simulink model "DSimulator_robot3GDL"  (Simulink 9.0)
settings: Solver=ode1  StartTime=0  StopTime=60  FixedStep=0.004  RelTol=1e-3  EnableMultiTasking=on
undefined symbols (not defined in the file or in its folder): Dinamic_ur10_3DOF, SimpleRobotPlotROS, Tau_JointSpace, Tau_OperationalSpace, TrajGen_JointSpace, TrajGen_OperationalSpace
libraries: simulink x3
settings Model: SuppressorTable=22 serialization::archive 11 0 6 0 0 0 11 0  Creator=E. Dean  LastModifiedBy=nirnai
settings DataIOCC: LimitDataPoints=on  SignalLoggingSaveFormat=ModelDataLogs
settings OptimizationCC: ExpressionDepthLimit=2147483647
settings DebuggingCC: SolverPrmCheckMsg=warning  FcnCallInpInsideContextMsg=warning  AllowSymbolicDim=off  StateNameClashWarn=warning
settings GRTTargetCC: GeneratePreprocessorConditionals=Disable all  CombineOutputUpdateFcns=off  GRTInterface=on
settings ConfigComp: CovSFcnEnable=off

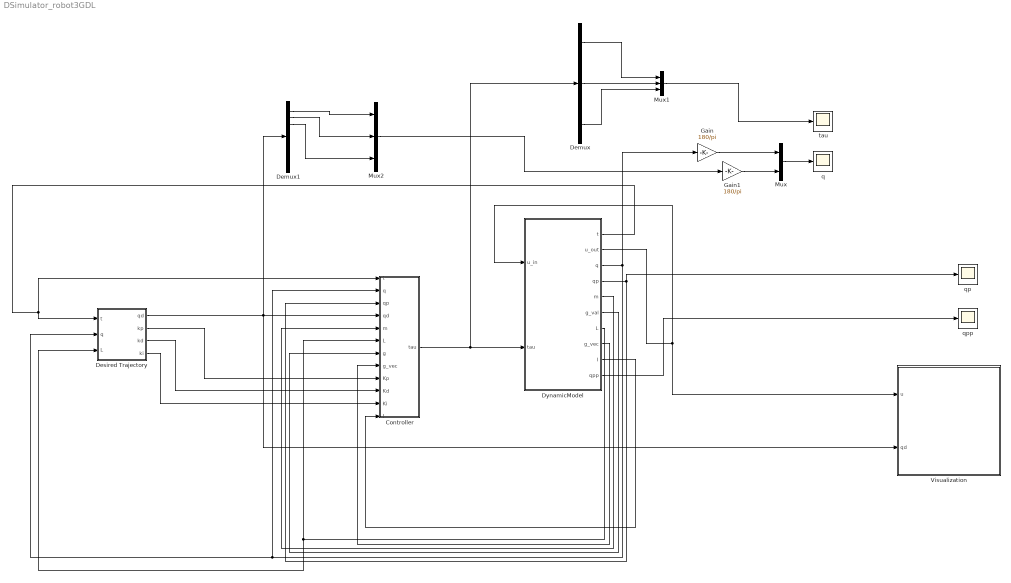
== system DSimulator_robot3GDL ==
  Controller : Subsystem
  Demux : Demux  Outputs=3
  Demux1 : Demux  Outputs=9
  Desired Trajectory : Subsystem
  DynamicModel : Subsystem
  Gain : Gain  Gain=180/pi
  Gain1 : Gain  Gain=180/pi
  Mux : Mux  Inputs=2
  Mux1 : Mux  Inputs=3
  Mux2 : Mux  Inputs=3
  Visualization : Subsystem
  q : Scope
  "qp " : Scope
  qpp : Scope
  tau : Scope
  wires:
  DynamicModel/2(u_out) -> DynamicModel/1(u_in), Visualization/1(u)
  DynamicModel/1("t ") -> Desired Trajectory/1(t), Controller/1(t)
  DynamicModel/3("q  ") -> Gain/1, Desired Trajectory/2(q), Controller/2(q)
  DynamicModel/4("qp ") -> Controller/3(qp), "qp "/1
  DynamicModel/5(m) -> Controller/5(m)
  DynamicModel/6(g_val) -> Controller/7(g)
  DynamicModel/7(L) -> Controller/6(L), Desired Trajectory/3(L)
  DynamicModel/8("g_vec ") -> Controller/8(g_vec)
  Controller/1(tau) -> Demux/1, DynamicModel/2(tau)
  Desired Trajectory/1(qd) -> Demux1/1, Visualization/2(qd), Controller/4(qd)
  Desired Trajectory/3(kd) -> Controller/10(Kd)
  Desired Trajectory/2("kp ") -> Controller/9(Kp)
  Desired Trajectory/4(ki) -> Controller/11(Ki)
  DynamicModel/9(I) -> Controller/12(I)
  Mux/1 -> q/1
  Gain/1 -> Mux/1
  Demux/1 -> Mux1/1
  Demux/2 -> Mux1/2
  Demux/3 -> Mux1/3
  Mux1/1 -> tau/1
  Demux1/1 -> Mux2/1
  Demux1/2 -> Mux2/2
  Demux1/3 -> Mux2/3
  Mux2/1 -> Gain1/1
  Gain1/1 -> Mux/2
  DynamicModel/10(qpp) -> qpp/1

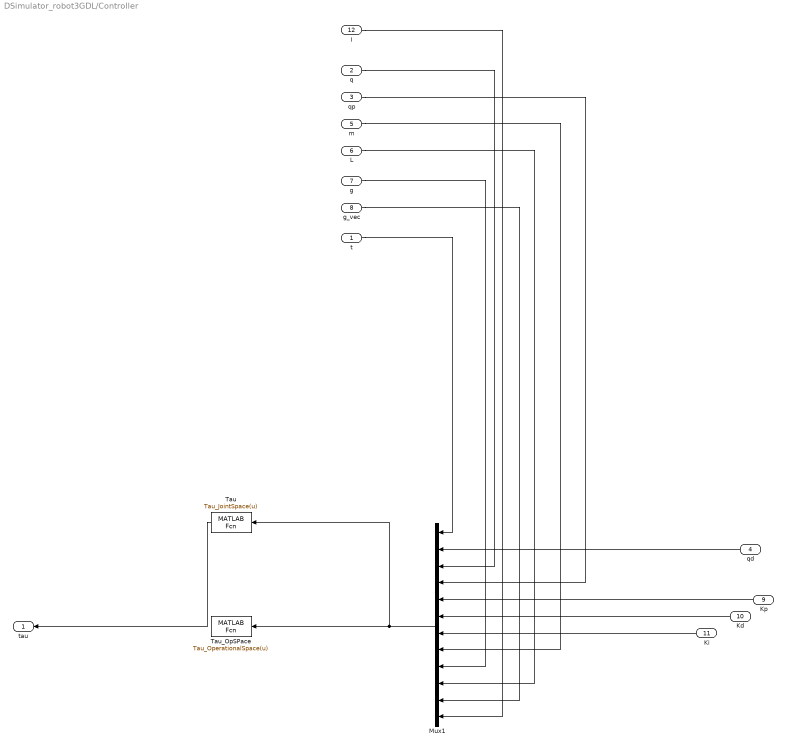
== system DSimulator_robot3GDL/Controller ==
  t : Inport
  q : Inport  Port=2
  qp : Inport  Port=3
  qd : Inport  Port=4
  m : Inport  Port=5
  L : Inport  Port=6
  g : Inport  Port=7
  g_vec : Inport  Port=8
  Kp : Inport  Port=9
  Kd : Inport  Port=10
  Ki : Inport  Port=11
  I : Inport  Port=12
  Mux1 : Mux  Inputs=12
  "Tau " : MATLABFcn  MATLABFcn=Tau_JointSpace(u)  OutputDimensions=3
  Tau_OpSPace : MATLABFcn  MATLABFcn=Tau_OperationalSpace(u)  OutputDimensions=3
  tau : Outport
  wires:
  t/1 -> Mux1/1
  L/1 -> Mux1/10
  q/1 -> Mux1/3
  qp/1 -> Mux1/4
  m/1 -> Mux1/8
  g_vec/1 -> Mux1/11
  Mux1/1 -> "Tau "/1, Tau_OpSPace/1
  Kd/1 -> Mux1/6
  I/1 -> Mux1/12
  g/1 -> Mux1/9
  Kp/1 -> Mux1/5
  Ki/1 -> Mux1/7
  qd/1 -> Mux1/2
  "Tau "/1 -> tau/1

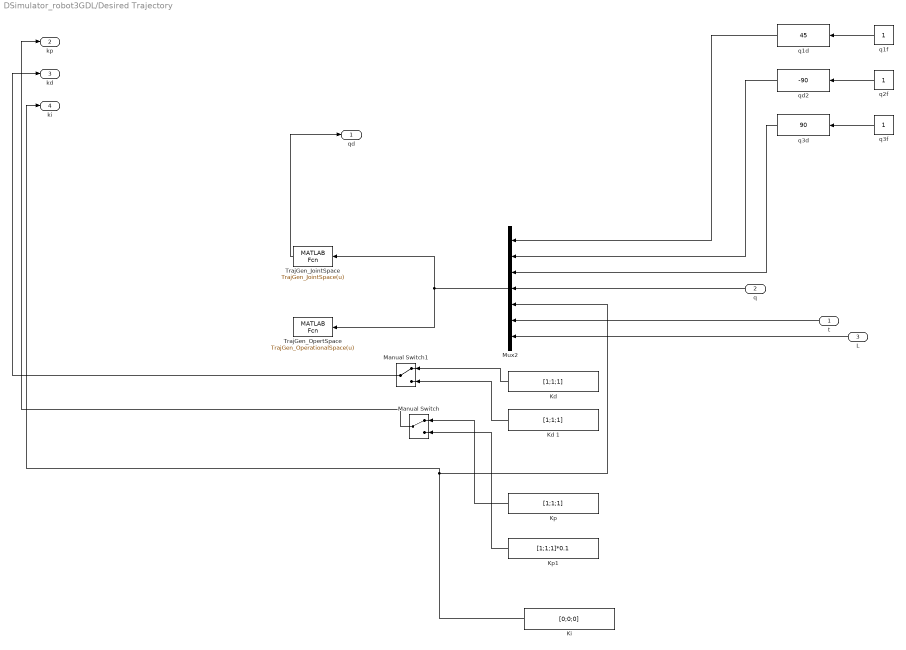
== system DSimulator_robot3GDL/Desired Trajectory ==
  t : Inport
  q : Inport  Port=2
  L : Inport  Port=3
  "Kd " : Constant  Value=[1;1;1]
  Kd 1 : Constant  Value=[1;1;1]
  Ki : Constant  Value=[0;0;0]
  Kp : Constant  Value=[1;1;1]
  Kp1 : Constant  Value=[1;1;1]*0.1
  Manual Switch : ManualSwitch
  Manual Switch1 : ManualSwitch
  Mux2 : Mux  Inputs=7
  TrajGen_JointSpace : MATLABFcn  MATLABFcn=TrajGen_JointSpace(u)  OutputDimensions=9
  TrajGen_OpertSpace : MATLABFcn  MATLABFcn=TrajGen_OperationalSpace(u)  OutputDimensions=21
  q1d : simulink/Math Operations/Slider Gain  gain=45  low=-180  high=180
  q1f : Constant
  q2f : Constant
  q3d : simulink/Math Operations/Slider Gain  gain=90  low=-180  high=180
  q3f : Constant
  qd2 : simulink/Math Operations/Slider Gain  gain=-90  low=-180  high=180
  qd : Outport
  "kp " : Outport  Port=2
  kd : Outport  Port=3
  ki : Outport  Port=4
  wires:
  Manual Switch1/1 -> kd/1
  Manual Switch/1 -> "kp "/1
  Ki/1 -> ki/1, Mux2/5
  t/1 -> Mux2/6
  q1f/1 -> q1d/1
  q2f/1 -> qd2/1
  q3f/1 -> q3d/1
  q1d/1 -> Mux2/1
  qd2/1 -> Mux2/2
  q3d/1 -> Mux2/3
  q/1 -> Mux2/4
  Mux2/1 -> TrajGen_OpertSpace/1, TrajGen_JointSpace/1
  L/1 -> Mux2/7
  TrajGen_JointSpace/1 -> qd/1
  Kp/1 -> Manual Switch/1
  Kp1/1 -> Manual Switch/2
  Kd 1/1 -> Manual Switch1/2
  "Kd "/1 -> Manual Switch1/1

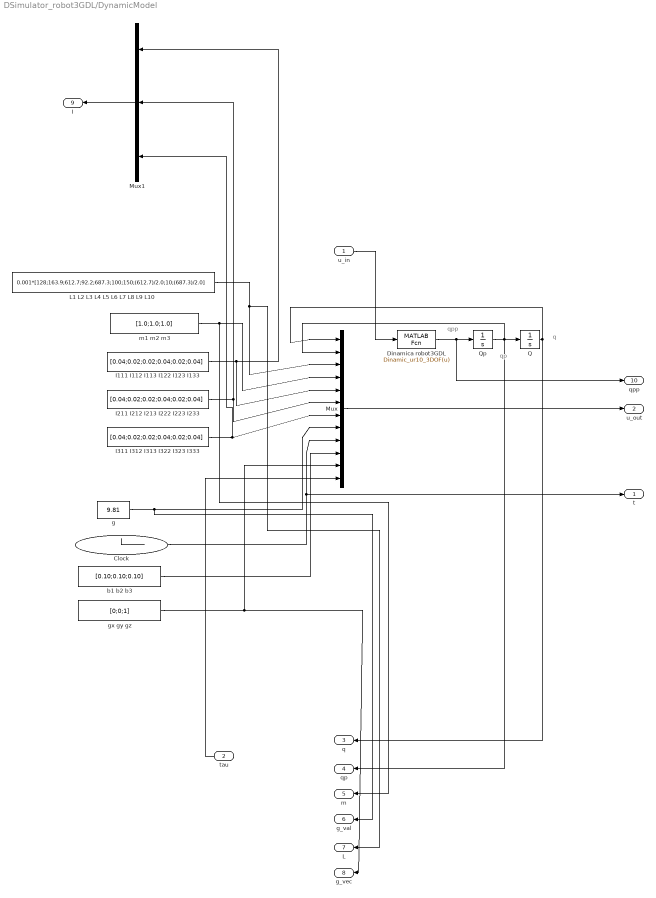
== system DSimulator_robot3GDL/DynamicModel ==
  note: q
  note: qp
  note: qpp
  u_in : Inport
  tau : Inport  Port=2
  Clock : Clock
  Dinamica robot3GDL : MATLABFcn  MATLABFcn=Dinamic_ur10_3DOF(u)  OutputDimensions=3
  I111 I112 I113 I122 I123 I133 : Constant  Value=[0.04;0.02;0.02;0.04;0.02;0.04]
  I211 I212 I213 I222 I223 I233 : Constant  Value=[0.04;0.02;0.02;0.04;0.02;0.04]
  I311 I312 I313 I322 I323 I333 : Constant  Value=[0.04;0.02;0.02;0.04;0.02;0.04]
  "L1 L2 L3 L4 L5 L6 L7 L8 L9 L10 " : Constant  Value=0.001*[128;163.9;612.7;92.2;687.3;100;150;(612.7)/2.0;10;(687.3)/2.0]  VectorParams1D=off
  Mux : Mux  Inputs=12
  Mux1 : Mux  Inputs=3
  Q : Integrator  InitialCondition=[0;-pi/2;0]
  Qp : Integrator  InitialCondition=[0;0;0]
  "b1 b2 b3 " : Constant  Value=[0.10;0.10;0.10]
  g : Constant  Value=9.81
  gx gy gz : Constant  Value=[0;0;1]
  "m1 m2 m3 " : Constant  Value=[1.0;1.0;1.0]
  "t " : Outport
  u_out : Outport  Port=2
  "q  " : Outport  Port=3
  "qp " : Outport  Port=4
  m : Outport  Port=5
  g_val : Outport  Port=6
  L : Outport  Port=7
  "g_vec " : Outport  Port=8
  I : Outport  Port=9
  qpp : Outport  Port=10
  wires:
  u_in/1 -> Dinamica robot3GDL/1
  I111 I112 I113 I122 I123 I133/1 -> Mux1/1, Mux/5
  I211 I212 I213 I222 I223 I233/1 -> Mux1/2, Mux/6
  I311 I312 I313 I322 I323 I333/1 -> Mux1/3, Mux/7
  "b1 b2 b3 "/1 -> Mux/10
  Mux/1 -> u_out/1
  Q/1 -> "q  "/1, Mux/1
  Qp/1 -> "qp "/1, Mux/2, Q/1
  "m1 m2 m3 "/1 -> m/1, Mux/4
  g/1 -> g_val/1, Mux/8
  "L1 L2 L3 L4 L5 L6 L7 L8 L9 L10 "/1 -> L/1, Mux/3
  Clock/1 -> "t "/1, Mux/9
  tau/1 -> Mux/12
  gx gy gz/1 -> "g_vec "/1, Mux/11
  Dinamica robot3GDL/1 -> qpp/1, Qp/1
  Mux1/1 -> I/1

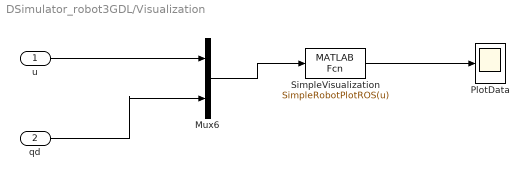
== system DSimulator_robot3GDL/Visualization ==
  u : Inport
  qd : Inport  Port=2
  Mux6 : Mux  Inputs=2
  PlotData : Scope
  SimpleVisualization : MATLABFcn  MATLABFcn=SimpleRobotPlotROS(u)  OutputDimensions=3
  wires:
  qd/1 -> Mux6/2
  u/1 -> Mux6/1
  SimpleVisualization/1 -> PlotData/1
  Mux6/1 -> SimpleVisualization/1
